simulink model "RTS_Template_ex4"  (R2020b)
settings: Solver=FixedStepAuto  StartTime=0  StopTime=inf  FixedStep=0.1  RelTol=1e-3
PreLoadFcn:
  | addpath(genpath('vis'));
StopFcn:
  | close all
libraries: simulink x1
settings Model: ODK_VersionTypeOld=V2.5  CpuAddresses=192.168.1.1:81  SimulationMode=external  Creator=Backbone  LastModifiedBy=Hendrik Streichhahn
settings DataIOCC: LimitDataPoints=on  SaveFormat=Array  SaveOutput=off  SaveTime=off  ReturnWorkspaceOutputs=off
settings OptimizationCC: LifeSpan=1
settings DebuggingCC: AllowSymbolicDim=off  SFUnexpectedBacktrackingDiag=warning  SFNoUnconditionalDefaultTransitionDiag=warning  SFExecutionAtInitializationDiag=none  ArithmeticOperatorsInVariantConditions=warning
settings HardwareCC: ProdBitPerPointer=32  ProdBitPerSizeT=32  ProdBitPerPtrDiffT=32  ProdWordSize=32  ProdHWDeviceType=Intel->x86-32 (Windows32)
settings ModelReferenceCC: PropagateSignalLabelsOutOfModel=off
settings SFSimCC: SimUseLocalCustomCode=off  CustomCodeUndefinedFunction=UseInterfaceOnly  SimTargetLang=C++
settings RTWCC: Description=Target for ODK capable S7-1500 Controllers based on Simulink Coder  SystemTargetFile=Target_1500S_V3_0_grt.tlc  GenCodeOnly=on  GenerateMakefile=off  TemplateMakefile=Target_1500S_V3_0_grt.tmf  GenerateReport=on  RTWVerbose=off  RTWUseLocalCustomCode=off  TargetLang=C++
settings CodeAppCC: ForceParamTrailComments=on  MaxIdLength=256  OperatorAnnotations=on  StateflowObjectComments=on  MATLABSourceComments=on
settings STFCustomTargetCC: ParMdlRefBuildCompliant=on  ConcurrentExecutionCompliant=off  CombineOutputUpdateFcns=on  CPPClassGenCompliant=off  GRTInterface=off  SystemTargetFile=Target_1500S_V3_0_grt.tlc
settings GRTTargetCC: TargetLangStandard=C89/C90 (ANSI)  CompOptLevelCompliant=off  ConcurrentExecutionCompliant=off  MatFileLogging=off  CPPClassGenCompliant=off  UseToolchainInfoCompliant=off  ExtModeStaticAlloc=on  ExtModeMexFile=mwsl_ext_comm_target1500s_v3  ExtModeMexArgs='192.168.0.1'
settings ConfigComp: CovMetricSettings=dw  CovSaveCumulativeToWorkspaceVar=on  CovSaveSingleToWorkspaceVar=on  CovExternalEMLEnable=off

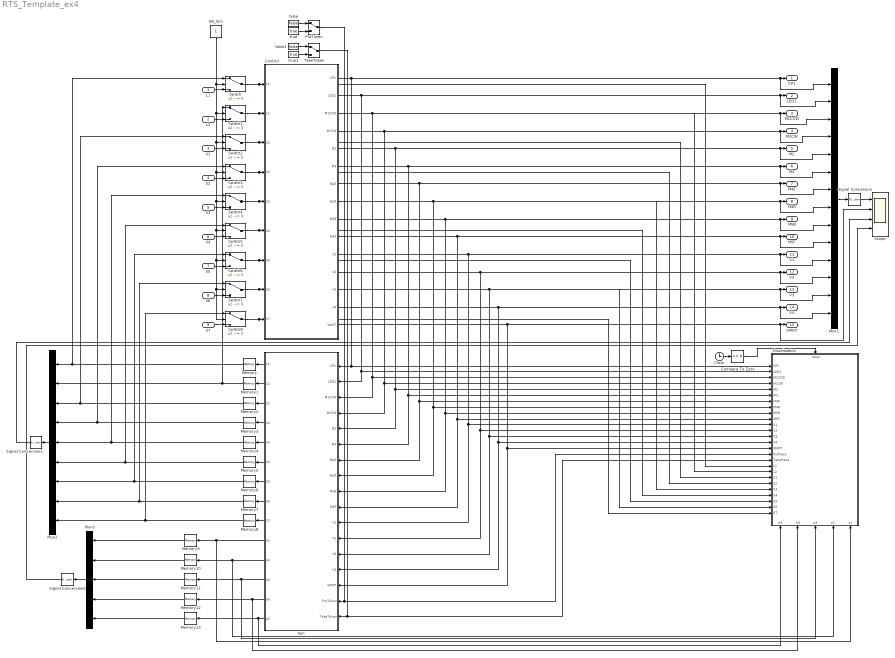
== system RTS_Template_ex4 ==
  L1 : Inport  OutDataTypeStr=boolean
  L2 : Inport  Port=2  OutDataTypeStr=boolean
  S1 : Inport  Port=3  OutDataTypeStr=boolean
  S2 : Inport  Port=4  OutDataTypeStr=boolean
  S3 : Inport  Port=5  OutDataTypeStr=boolean
  S4 : Inport  Port=6  OutDataTypeStr=boolean
  S5 : Inport  Port=7  OutDataTypeStr=boolean
  S6 : Inport  Port=8  OutDataTypeStr=boolean
  S7 : Inport  Port=9  OutDataTypeStr=boolean
  Clock : Clock
  Compare To Zero : simulink/Logic and Bit Operations/Compare To Zero  relop=<=  OutDataTypeStr=boolean
  Control : Stateflow chart  TreatAsAtomicUnit=on
  EN_Sim : Constant
  Memory : Memory  InitialCondition=1
  Memory1 : Memory  InitialCondition=1
  Memory{2..13} (12 alike) : Memory
  Mux1 : Mux  Inputs=14
  Mux2 : Mux  Inputs=9
  Mux3 : Mux  Inputs=5
  PutToken : ManualSwitch
  Scope : Scope  NumInputPorts=4
  Signal Conversion : SignalConversion  OverrideOpt=off
  Signal Conversion1 : SignalConversion  OverrideOpt=off
  Signal Conversion2 : SignalConversion  OverrideOpt=off
  Sim : Stateflow chart  TreatAsAtomicUnit=on
  Switch{,1..8} (9 alike) : Switch  Criteria=u2 ~= 0  Threshold=1
  TakeToken : ManualSwitch
  "Visualisation " : Stateflow chart  TreatAsAtomicUnit=on
      settings: PortSchema="{\"entries\":[{\"content\":{\"sides\":[{\"content\":{\"connectorIds\":[\"In11\",\"In12\",\"In13\",\"In14\",\"In15\",\"In16\",\"In17\",\"In18\",\"In19\",\"In20\",\"In21\",\"In22\",\"In23\",\"In24\",\"In25\",\"In26\",\"In27\",\"In2\",\"In3\",\"In4\",\"In5\",\"In6\",\"In7\",\"In8\",\"In9\",\"In10\"]},\"type\":\"ConnectorPlacement.EquallySpacedRectSide\",\"uuid\":\"2c00268f-01f2-48a9-bb45-08f3cdafe229\"},{\"content\":{\"connectorIds\":[],\"side\":\"RIGHT\"},\"type\":\"ConnectorPlacement.EquallySpacedRectSide\",\"uuid\":\"314ddca5-10ac-44b2-bea6-2b443d6fccb4\"},{\"content\":{\"connectorIds\":[\"In1\"],\"side\":\"TOP\"},\"type\":\"ConnectorPlacement.EquallySpacedRectSide\",\"uuid\":\"6c22254f-ebe8-4a94-a5e1-578889e215de\"},{\"content\":{\"connectorIds\":[\"In32\",\"In31\",\"In30\",\"In29\",\"In28\"],\"side\":\"BOTTOM\"},\"type\":\"ConnectorPlacement.EquallySpacedRectSide\",\"uuid\":\"478d9fd1-a645-41f2-bcdf-af5e15a67641\"},{\"content\":{\"connectorIds\":[],\"side\":\"HIDDEN\"},\"type\":\"ConnectorPlacement.EquallySpacedRectSide\",\"uuid\":\"cf51fa7f-a8e0-4e0e-af76-c02387c93b0b\"}]},\"type\":\"ConnectorPlacement.EquallySpacedConnector\",\"uuid\":\"84175e4e-5022-4463-b529-e7ba99fa8ea4\"}],\"packageUris\":[\"http://schema.mathworks.com/mf0/Connector/R2020b\"],\"version\":\"1.0\"}"
  false : Constant  Value=false
  false1 : Constant  Value=false
  true : Constant  Value=true
  true1 : Constant  Value=true
  CP1 : Outport  OutDataTypeStr=boolean  VectorParamsAs1DForOutWhenUnconnected=off
  LED1 : Outport  Port=2  OutDataTypeStr=boolean  VectorParamsAs1DForOutWhenUnconnected=off
  M1CCW : Outport  Port=3  OutDataTypeStr=boolean  VectorParamsAs1DForOutWhenUnconnected=off
  M1CW : Outport  Port=4  OutDataTypeStr=boolean  VectorParamsAs1DForOutWhenUnconnected=off
  M2 : Outport  Port=5  OutDataTypeStr=boolean  VectorParamsAs1DForOutWhenUnconnected=off
  M3 : Outport  Port=6  OutDataTypeStr=boolean  VectorParamsAs1DForOutWhenUnconnected=off
  M4E : Outport  Port=7  OutDataTypeStr=boolean  VectorParamsAs1DForOutWhenUnconnected=off
  M4R : Outport  Port=8  OutDataTypeStr=boolean  VectorParamsAs1DForOutWhenUnconnected=off
  M5B : Outport  Port=9  OutDataTypeStr=boolean  VectorParamsAs1DForOutWhenUnconnected=off
  M5F : Outport  Port=10  OutDataTypeStr=boolean  VectorParamsAs1DForOutWhenUnconnected=off
  V1 : Outport  Port=11  OutDataTypeStr=boolean  VectorParamsAs1DForOutWhenUnconnected=off
  V2 : Outport  Port=12  OutDataTypeStr=boolean  VectorParamsAs1DForOutWhenUnconnected=off
  V3 : Outport  Port=13  OutDataTypeStr=boolean  VectorParamsAs1DForOutWhenUnconnected=off
  V4 : Outport  Port=14  OutDataTypeStr=boolean  VectorParamsAs1DForOutWhenUnconnected=off
  VMOT : Outport  Port=15  OutDataTypeStr=uint8  VectorParamsAs1DForOutWhenUnconnected=off
  wires:
  Mux1/1 -> Signal Conversion/1
  Signal Conversion/1 -> Scope/1
  Control/1(CP1) -> "Visualisation "/11(CP1), Sim/1(CP1), Mux1/1, CP1/1
  Control/2(LED1) -> Sim/2(LED1), "Visualisation "/12(LED1), Mux1/2, LED1/1
  Control/3(M1CCW) -> Sim/3(M1CCW), "Visualisation "/13(M1CCW), Mux1/3, M1CCW/1
  Control/5(M2) -> Sim/5(M2), "Visualisation "/15(M2), Mux1/5, M2/1
  Control/6(M3) -> Sim/6(M3), "Visualisation "/16(M3), Mux1/6, M3/1
  Control/7(M4E) -> Sim/7(M4E), "Visualisation "/17(M4E), Mux1/7, M4E/1
  Control/8(M4R) -> Sim/8(M4R), "Visualisation "/18(M4R), Mux1/8, M4R/1
  Control/9(M5B) -> Sim/9(M5B), "Visualisation "/19(M5B), Mux1/9, M5B/1
  Control/10(M5F) -> Sim/10(M5F), "Visualisation "/20(M5F), Mux1/10, M5F/1
  Control/11(V1) -> Sim/11(V1), "Visualisation "/21(V1), Mux1/11, V1/1
  Control/12(V2) -> Sim/12(V2), "Visualisation "/22(V2), Mux1/12, V2/1
  Control/13(V3) -> Sim/13(V3), "Visualisation "/23(V3), Mux1/13, V3/1
  Control/14(V4) -> Sim/14(V4), "Visualisation "/24(V4), Mux1/14, V4/1
  Control/15(VMOT) -> Sim/15(VMOT), "Visualisation "/25(VMOT), Scope/2, VMOT/1
  Switch/1 -> "Visualisation "/2(L1), Control/1(L1)
  Switch1/1 -> "Visualisation "/3(L2), Control/2(L2)
  Switch2/1 -> "Visualisation "/4(S1), Control/3(S1)
  Switch3/1 -> "Visualisation "/5(S2), Control/4(S2)
  Switch4/1 -> "Visualisation "/6(S3), Control/5(S3)
  Switch5/1 -> "Visualisation "/7(S4), Control/6(S4)
  Switch6/1 -> "Visualisation "/8(S5), Control/7(S5)
  Switch7/1 -> "Visualisation "/9(S6), Control/8(S6)
  Switch8/1 -> "Visualisation "/10(S7), Control/9(S7)
  EN_Sim/1 -> Switch8/2, Switch7/2, Switch6/2, Switch5/2, Switch4/2, Switch3/2, Switch2/2, Switch1/2, Switch/2
  Sim/1(L1) -> Memory/1
  Sim/2(L2) -> Memory1/1
  Sim/3(S1) -> Memory2/1
  Sim/4(S2) -> Memory3/1
  Sim/5(S3) -> Memory4/1
  Sim/6(S4) -> Memory5/1
  Sim/7(S5) -> Memory6/1
  Sim/8(S6) -> Memory7/1
  Sim/9(S7) -> Memory8/1
  Memory/1 -> Switch/1, Mux2/1
  Memory1/1 -> Mux2/2, Switch1/1
  Memory2/1 -> Mux2/3, Switch2/1
  Memory3/1 -> Mux2/4, Switch3/1
  Memory4/1 -> Mux2/5, Switch4/1
  Memory5/1 -> Mux2/6, Switch5/1
  Memory6/1 -> Mux2/7, Switch6/1
  Memory7/1 -> Mux2/8, Switch7/1
  Memory8/1 -> Mux2/9, Switch8/1
  false/1 -> PutToken/1
  true/1 -> PutToken/2
  PutToken/1 -> "Visualisation "/26(PutPiece), Sim/16(PutToken)
  true1/1 -> TakeToken/2
  false1/1 -> TakeToken/1
  TakeToken/1 -> "Visualisation "/27(TakePiece), Sim/17(TakeToken)
  Mux2/1 -> Signal Conversion1/1
  Signal Conversion1/1 -> Scope/3
  Compare To Zero/1 -> "Visualisation "/1(reset)
  Clock/1 -> Compare To Zero/1
  Control/4(M1CW) -> Sim/4(M1CW), "Visualisation "/14(M1CW), Mux1/4, M1CW/1
  Sim/13(p4) -> "Visualisation "/31(p4), Memory12/1
  Sim/12(p3) -> "Visualisation "/30(p3), Memory11/1
  Sim/11(p2) -> "Visualisation "/29(p2), Memory10/1
  Sim/10(p1) -> "Visualisation "/28(p1), Memory9/1
  Memory9/1 -> Mux3/1
  Memory10/1 -> Mux3/2
  Memory11/1 -> Mux3/3
  Memory12/1 -> Mux3/4
  Mux3/1 -> Signal Conversion2/1
  Signal Conversion2/1 -> Scope/4
  L1/1 -> Switch/3
  L2/1 -> Switch1/3
  S1/1 -> Switch2/3
  S2/1 -> Switch3/3
  S3/1 -> Switch4/3
  S4/1 -> Switch5/3
  S5/1 -> Switch6/3
  S6/1 -> Switch7/3
  S7/1 -> Switch8/3
  Memory13/1 -> Mux3/5
  Sim/14(p5) -> "Visualisation "/32(p5), Memory13/1

== stateflow chart RTS_Template_ex4/Sim ==
  state Oven [parallel]
    settings: executionOrder=2
    state M4EControl
      entry:S5=(p1==1)
      entry:S6=(p1==0)
      entry:L2= (tokenInOven & p1< 0.25)
    state MoveIn
      entry:p1=min(p1+0.05, 1)
      entry:S5=(p1==1.0)
      entry:L2= (tokenInOven & p1 < 0.25)
    state MoveOut
      entry:p1=max(p1-0.05, 0)
      entry:S6=(p1==0.0)
      entry:L2= (tokenInOven & p1< 0.25)
    state Init
      entry:~tokenInOven
    MoveIn -> MoveIn [order 2] : [after(0.2,sec)]
    M4EControl -> MoveIn [order 1] : [M4E]
    MoveIn -> M4EControl [order 1] : [~M4E]
    M4EControl -> M4EControl [order 3] : [PutToken]{~L2, tokenInOven}
    Init -> M4EControl
    MoveOut -> M4EControl [order 1] : [~M4R]
    M4EControl -> MoveOut [order 2] : [M4R]
    MoveOut -> MoveOut [order 2] : [after(0.2,sec)]
    (default) -> Init
  state General [parallel]
    en:L1=true;
    en:L2=true;
    en:S1=false;
    en:S2=false;
    en:S3=false;
    en:S4=false;
    en:S5=false;
    en:S6=false;
    en:S7=false;
    en:p1=0.5;
    en:p2=0.5;
    en:p3=0.5;
    en:p4=0.5;
    en:p5=0;
    settings: executionOrder=1
  state Gripper [parallel]
    settings: executionOrder=3
    state GripperMoveRight [parallel]
      settings: executionOrder=1
      state M5B_Wait
        entry: S4 = (p2==1.0)
      state M5B_Move
        entry: p2=min(p2+0.05,1)
        entry: S4 = (p2==1.0)
      (default) -> M5B_Wait
      M5B_Wait -> Gripper.GripperMoveRight.M5B_Move [order 1] : [M5B]
      Gripper.GripperMoveRight.M5B_Move -> M5B_Wait [order 1] : [~M5B]
      M5B_Wait -> M5B_Wait [order 2] : after(0.2,sec)
      Gripper.GripperMoveRight.M5B_Move -> Gripper.GripperMoveRight.M5B_Move [order 2] : after(0.2,sec)
    state takeToken [parallel]
      settings: executionOrder=3
      state wait
      state take
        entry:~tokenInOven
      state waitArm
      (default) -> wait
      take -> wait : after(0.2,sec)
      waitArm -> take : after(1.8,sec)
      wait -> waitArm : [S7&V1&V2]
    state GripperMoveLeft [parallel]
      settings: executionOrder=2
      state M5F_Wait
        entry: S7 = (p2==1.0)
      state M5B_Move
        entry: p2=max(p2-0.05,1)
        entry: S7 = (p2==1.0)
      (default) -> M5F_Wait
      M5F_Wait -> Gripper.GripperMoveLeft.M5B_Move [order 1] : [M5F]
      Gripper.GripperMoveLeft.M5B_Move -> M5F_Wait [order 1] : [~M5F]
      M5F_Wait -> M5F_Wait [order 2] : after(0.2,sec)
      Gripper.GripperMoveLeft.M5B_Move -> Gripper.GripperMoveLeft.M5B_Move [order 2] : after(0.2,sec)
  state Conveyor [parallel]
    settings: executionOrder=5
    state L1Free
      en:L1=true;
    state Extend
      en:p5=min(p5+0.05,1);
    state WaitConveyOff
    state L1Interrupted
      en:L1=false;
    state TakeComplete
      en:L1=true;
    state WaitTakeComplete
      ex:p5=0;
    (default) -> L1Free
    L1Free -> Extend [order 1] : [M2]
    Extend -> L1Free [order 1] : [~M2]
    Extend -> Extend [order 2] : after(0.2,sec)
    Extend -> L1Interrupted [order 3] : [p5>=1]
    WaitConveyOff -> L1Free : [~M2]
    L1Free -> L1Interrupted [order 2] : [p5>=1]
    TakeComplete -> WaitConveyOff : [M2]
    L1Interrupted -> WaitTakeComplete : [TakeToken]
    WaitTakeComplete -> TakeComplete : [~TakeToken]
  state Turntable [parallel]
    settings: executionOrder=4
    state MoveM1CCW [parallel]
      settings: executionOrder=1
      state M1CCW_Wait
      state M1CCW_Move
        entry:p3=min(p3+0.05,1)
      M1CCW_Move -> M1CCW_Move [order 2] : after(0.2,sec)
      (default) -> M1CCW_Wait
      M1CCW_Wait -> M1CCW_Move : [M1CCW]
      M1CCW_Move -> M1CCW_Wait [order 1] : [~M1CCW]
    state ControlS1 [parallel]
      settings: executionOrder=3
      state control
        entry:S1=(p3==0)
      (default) -> Turntable.ControlS1.control
      Turntable.ControlS1.control -> Turntable.ControlS1.control : after(0.1,sec)
    state ControlS3 [parallel]
      settings: executionOrder=4
      state control
        entry:S3=(p3>0.5)&(p3<0.75)
      (default) -> Turntable.ControlS3.control
      Turntable.ControlS3.control -> Turntable.ControlS3.control : after(0.1,sec)
    state MoveM1CW [parallel]
      settings: executionOrder=2
      state M1CW_Wait
      state M1CW_Move
        entry: p3=max(p3-0.05,1)
      (default) -> M1CW_Wait
      M1CW_Move -> M1CW_Move [order 2] : after(0.2,sec)
      M1CW_Wait -> M1CW_Move : [M1CW]
      M1CW_Move -> M1CW_Wait [order 1] : [~M1CW]
    state ControlS2 [parallel]
      settings: executionOrder=5
      state control
        entry:S2=(p3==1)
      (default) -> Turntable.ControlS2.control
      Turntable.ControlS2.control -> Turntable.ControlS2.control : after(0.1,sec)
    state MoveV4 [parallel]
      settings: executionOrder=6
      state extend
        entry: p4=min(p4+0.2,1)
      state retract
        entry: p4=max(p4-0.2,0)
      (default) -> retract
      retract -> extend [order 1] : [V4]
      extend -> retract [order 1] : [~V4]
      retract -> retract [order 2] : after(0.2,sec)
      extend -> extend [order 2] : after(0.2,sec)
  data: CP1 input; LED1 input; M1CCW input; M1CW input; M2 input; M3 input; M4E input; M4R input; M5B input; M5F input; V1 input; V2 input; V3 input; V4 input; VMOT input; L1 output; L2 output; S1 output; S2 output; S3 output; S4 output; S5 output; S6 output; S7 output; PutToken input; TakeToken input; p1 output; p2 output; p3 output; p4 output; p5 output; tokenInOven local boolean size=1 =false

== stateflow chart RTS_Template_ex4/Visualisation  ==
  note: Do not change!
  state Init
    en: ml.vis=ml.createVis();
  state Update
    en: ml.vis=ml.updateVis(ml.vis,reset,L1,L2,S1,S2,S3,S4,S5,S6,S7,CP1,LED1,M1CCW,M1CW,M2,M3,M4E,M4R,M5B,M5F,V1,V2,V3,V4,VMOT,PutPiece,TakePiece,p1,p2,p3,p4,p5);
  (default) -> Init
  Init -> Init [order 1] : [reset]
  Update -> Init [order 2] : [reset]
  Init -> Update [order 2] : after(0.1,sec)[~reset]
  Update -> Update [order 1] : after(0.1,sec)
  data: reset input; L1 input; L2 input; S1 input; S2 input; S3 input; S4 input; S5 input; S6 input; S7 input; CP1 input; LED1 input; M1CCW input; M1CW input; M2 input; M3 input; M4E input; M4R input; M5B input; M5F input; V1 input; V2 input; V3 input; V4 input; VMOT input; PutPiece input; TakePiece input; p1 input; p2 input; p3 input; p4 input; p5 input

== stateflow chart RTS_Template_ex4/Control ==
  state General [parallel]
    en: CP1=false;
    en: LED1=false;
    en:  M1CCW=false;
    en:  M1CW=false;
    en:  M2=false;
    en:  M3=false;
    en:  M4E=false;
    en:  M4R=false;
    en:  M5B=false;
    en: M5F=false;
    en: V1=false;
    en: V2=false;
    en: V3=false;
    en: V4=false;
    en: VMOT=uint8(255);
    settings: executionOrder=1
  state Oven [parallel]
    settings: executionOrder=2
    state Init
      entry:CP1,V3
      during: M4R
    state readyPos
      entry: ~OvenHasToken
    state waitForTake
      entry: OvenHasToken
    state tokenInput
      during: M4E
      exit: ~V3
    state heating
      during: LED1
    state tokenOutput
      entry: V3
      during: M4R
    (default) -> Oven.Init
    Oven.Init -> readyPos : [S6]
    Oven.waitForTake -> readyPos : [L2]
    readyPos -> tokenInput : [~L2]
    tokenOutput -> Oven.waitForTake : [S6]
    tokenInput -> heating : [S5]
    heating -> tokenOutput : [after(5,sec)]
  state Gripper [parallel]
    settings: executionOrder=3
    state ungrip
      entry:TurnTablePut,~V1
    state loweringArm1
      entry:V2
    state Init
      entry:V2
      during:M5F
    state turntableWait
    state armUp1
      entry:~V2
    state ready
    state gotoTurntable
      during:M5F
    state gotoOven
      during: M5B
    state loweringArm
      entry:V2
    state VacuumGrip
      entry: V1
    state armUp
      entry: ~V2
    (default) -> Gripper.Init
    ungrip -> armUp1 : after(2,sec)
    loweringArm1 -> ungrip : after(2,sec)
    turntableWait -> loweringArm1 : [S1]
    Gripper.Init -> Gripper.ready : [S4]
    gotoTurntable -> turntableWait : [S4]
    armUp1 -> Gripper.ready : after(2,sec)
    Gripper.ready -> gotoOven : [OvenHasToken]
    armUp -> gotoTurntable : [after(2,sec)]
    gotoOven -> loweringArm : [S7]
    loweringArm -> VacuumGrip : after(2,sec)
    VacuumGrip -> armUp : after(2,sec)
  state Conveyor [parallel]
    settings: executionOrder=5
    state Init
      entry: ~ConveyorFree
      during: M2
    state waitForTake
    state ready
      during: ConveyorFree
    state transport
      during: M2
      exit: ~ConveyorPut
    (default) -> Conveyor.Init
    Conveyor.Init -> Conveyor.ready : [L1]
    Conveyor.waitForTake -> Conveyor.ready : [L1]
    transport -> Conveyor.waitForTake : [~L1]
    Conveyor.ready -> transport : [ConveyorPut]
  state Turntable [parallel]
    settings: executionOrder=4
    state Init
      during: M1CCW
    state pushToken
      during: V4
    state WaitConveyorFree
    state ready
    state MoveToConveyor
      during: M1CW
    state moveToSaw
      entry: ~TurnTablePut
      during: M1CW
    state sawing
      during: M3
    (default) -> Turntable.Init
    pushToken -> Turntable.Init : after(2,sec)
    WaitConveyorFree -> pushToken : [L1]
    Turntable.Init -> Turntable.ready : [S1]
    MoveToConveyor -> WaitConveyorFree : [S2]
    Turntable.ready -> moveToSaw : [TurnTablePut]
    sawing -> MoveToConveyor : after(2,sec)
    moveToSaw -> sawing : [S3]
  data: L1 input; L2 input; S1 input; S2 input; S3 input; S4 input; S5 input; S6 input; S7 input; CP1 output; LED1 output; M1CCW output; M1CW output; M2 output; M3 output; M4E output; M4R output; M5B output; M5F output; V1 output; V2 output; V3 output; V4 output; VMOT output; OvenHasToken local boolean =false; TurnTablePut local boolean =false; ConveyorFree local boolean =true; ConveyorPut local boolean =false
